simulink model "TRASFUNCTION"  (R2025b)
settings: Solver=VariableStepAuto  StartTime=0.0  StopTime=50.0  RelTol=1e-3
settings Model: Creator=Roshan jena  LastModifiedBy=Roshan jena

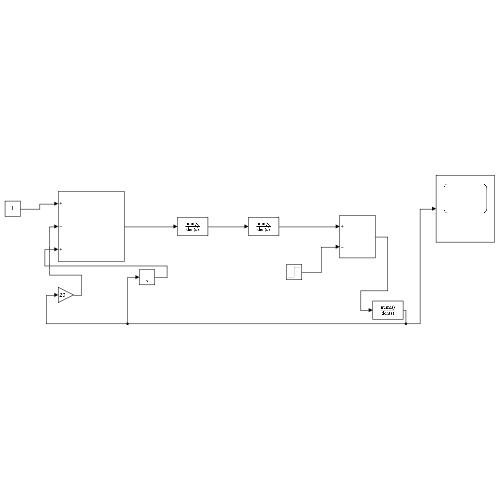
[thumbnail: Simulink's stored preview of the top-level diagram]
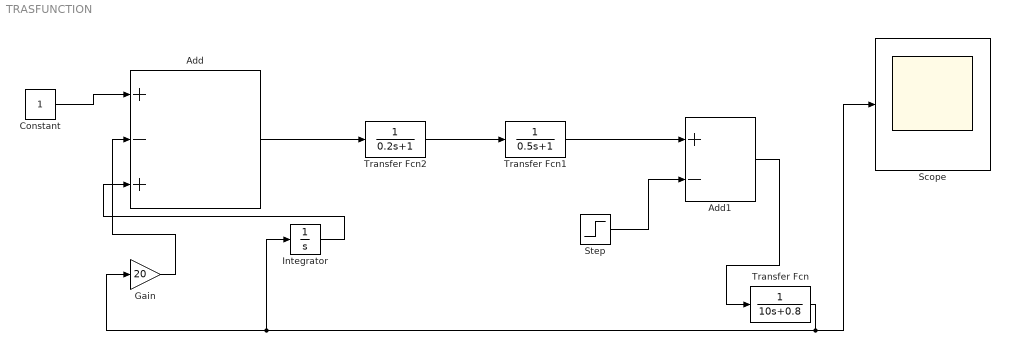
== system TRASFUNCTION ==
  Add : Sum  Inputs=+-+
  Add1 : Sum  Inputs=+-
  Constant : Constant
  Gain : Gain  Gain=20
  Integrator : Integrator
  Scope : Scope
  Step : Step  After=0.2  SampleTime=1
  Transfer Fcn : TransferFcn  Denominator=[10 0.8]
  Transfer Fcn1 : TransferFcn  Denominator=[0.5 1]
  Transfer Fcn2 : TransferFcn  Denominator=[0.2 1]
  wires:
  Add/1 -> Transfer Fcn2/1
  Transfer Fcn2/1 -> Transfer Fcn1/1
  Constant/1 -> Add/1
  Transfer Fcn1/1 -> Add1/1
  Step/1 -> Add1/2
  Add1/1 -> Transfer Fcn/1
  Transfer Fcn/1 -> Scope/1, Integrator/1, Gain/1
  Gain/1 -> Add/2
  Integrator/1 -> Add/3
